simulink model "platform_B1"  (R2021b)
settings: Solver=ode4  StartTime=0.0  StopTime=time_end  FixedStep=Ts  RelTol=1e-3  EnableMultiTasking=on
settings Model: Creator=Furao  LastModifiedBy=Furao
settings SolverCC: AlgebraicLoopSolver=TrustRegion
settings DataIOCC: LimitDataPoints=on  SaveFormat=Array  ReturnWorkspaceOutputs=off  SignalLoggingName=sigsOut
settings DebuggingCC: SaveWithParameterizedLinksMsg=none  UnderspecifiedInitializationDetection=Classic  MergeDetectMultiDrivingBlocksExec=none  SignalResolutionControl=TryResolveAllWithWarning  MultiTaskDSMMsg=warning  MultiTaskCondExecSysMsg=none  SFMachineParentedDataDiag=warning  ArithmeticOperatorsInVariantConditions=warning
settings HardwareCC: ProdBitPerPointer=32  ProdBitPerSizeT=32  ProdBitPerPtrDiffT=32  ProdLargestAtomicFloat=None  ProdIntDivRoundTo=Undefined  ProdEndianess=Unspecified  ProdWordSize=32  ProdHWDeviceType=32-bit Generic  TargetUnknown=on
settings ModelReferenceCC: PropagateSignalLabelsOutOfModel=off
settings SFSimCC: SimUseLocalCustomCode=off  CustomCodeUndefinedFunction=UseInterfaceOnly
settings RTWCC: RTWUseLocalCustomCode=off
settings CodeAppCC: StateflowObjectComments=on
settings GRTTargetCC: TargetLangStandard=C89/C90 (ANSI)  CombineOutputUpdateFcns=off  GRTInterface=on
settings ConfigComp: CovMetricSettings=dw  CovSaveCumulativeToWorkspaceVar=on  CovSaveSingleToWorkspaceVar=on  CovExternalEMLEnable=off

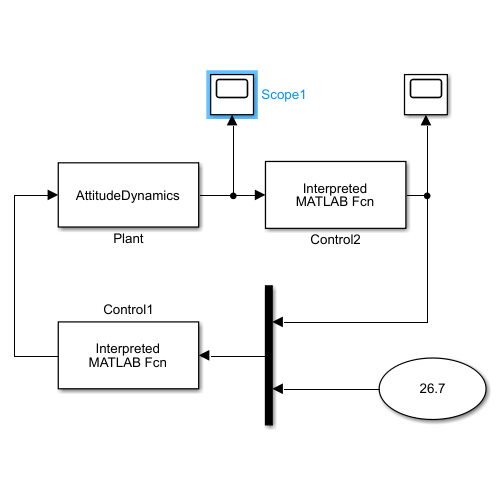
[thumbnail: Simulink's stored preview of the top-level diagram]
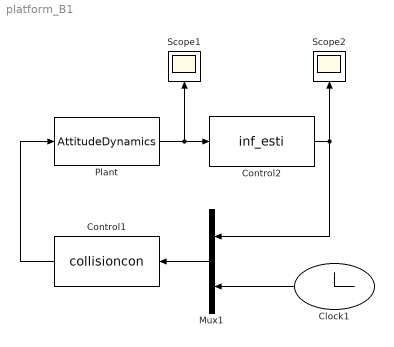
== system platform_B1 ==
  Clock1 : Clock
  Control1 : MATLABFcn  MATLABFcn=collisioncon
  Control2 : MATLABFcn  MATLABFcn=inf_esti
  Mux1 : Mux  Inputs=2
  Plant : S-Function  FunctionName=AttitudeDynamics  SFunctionDeploymentMode=off  EnableBusSupport=off
  Scope1 : Scope
  Scope2 : Scope
  wires:
  Mux1/1 -> Control1/1
  Clock1/1 -> Mux1/2
  Control1/1 -> Plant/1
  Plant/1 -> Control2/1, Scope1/1
  Control2/1 -> Scope2/1, Mux1/1
